simulink model "airspeed_from_pitch_loop"  (R2019a)
settings: Solver=VariableStepAuto  StartTime=0.0  StopTime=1000  RelTol=1e-3
undefined symbols (not defined in the file or in its folder): AP, trans_func
settings Model: Creator=nikhil  LastModifiedBy=VTOL_HYD

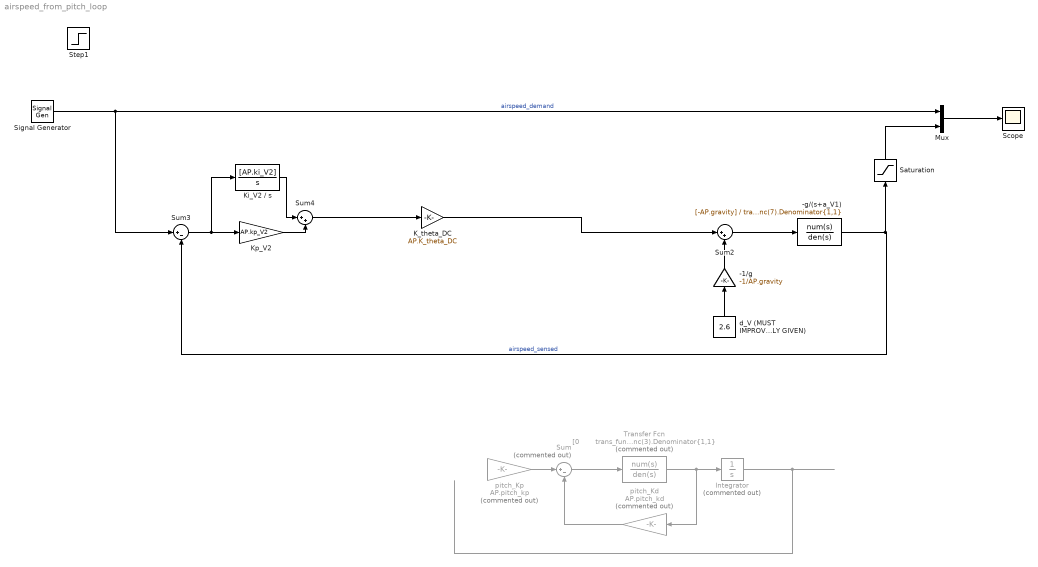
== system airspeed_from_pitch_loop ==
  -1/g : Gain  Gain=-1/AP.gravity
  -g/(s+a_V1) : TransferFcn  Numerator=[-AP.gravity]  Denominator=trans_func(7).Denominator{1,1}
  Integrator : Integrator  Commented=on
  "K_theta_DC " : Gain  Gain=AP.K_theta_DC
  Ki_V2 / s : TransferFcn  Numerator=[AP.ki_V2]  Denominator=[1 0]
  Kp_V2 : Gain  Gain=AP.kp_V2
  Mux : Mux  Inputs=2
  Saturation : Saturate  UpperLimit=200  LowerLimit=-200
  Scope : Scope
  Signal Generator : SignalGenerator  WaveForm=sawtooth  Amplitude=45  Frequency=.1  Units=rad/sec
  Step1 : Step  Time=8  After=35  SampleTime=0
  Sum : Sum  Commented=on  Inputs=|+-
  Sum2 : Sum  Inputs=|++
  Sum3 : Sum  Inputs=|+-
  Sum4 : Sum  Inputs=|++
  Transfer Fcn : TransferFcn  Commented=on  Numerator="[0        trans_func(3).Numerator{1,1}(3)       0]"  Denominator=trans_func(3).Denominator{1,1}
  d_V (MUST IMPROVE! FORMULA NOT FULLY GIVEN) : Constant  Value=2.6
  pitch_Kd : Gain  Commented=on  Gain=AP.pitch_kd
  pitch_Kp : Gain  Commented=on  Gain=AP.pitch_kp
  wires:
  -g/(s+a_V1)/1 -> Saturation/1, Sum3/2  "airspeed_sensed"
  Mux/1 -> Scope/1
  Sum4/1 -> "K_theta_DC "/1
  Ki_V2 / s/1 -> Sum4/1
  Kp_V2/1 -> Sum4/2
  Signal Generator/1 -> Sum3/1, Mux/1  "airspeed_demand"
  Sum3/1 -> Ki_V2 / s/1, Kp_V2/1
  -1/g/1 -> Sum2/2
  d_V (MUST IMPROVE! FORMULA NOT FULLY GIVEN)/1 -> -1/g/1
  Sum2/1 -> -g/(s+a_V1)/1
  Saturation/1 -> Mux/2
  Integrator/1 -> ?
  ? -> pitch_Kp/1
  pitch_Kd/1 -> Sum/2
  Sum/1 -> Transfer Fcn/1
  pitch_Kp/1 -> Sum/1
  Transfer Fcn/1 -> pitch_Kd/1, Integrator/1
  "K_theta_DC "/1 -> Sum2/1
